simulink library "ParsingLibrary"  (Simulink 8.2)
settings: Solver=ode45  StartTime=0.0  StopTime=10.0  RelTol=1e-3
undefined symbols (not defined in the file): Indicies
libraries: simulink x1
settings Model: Creator=Scott  LastModifiedBy=leidos

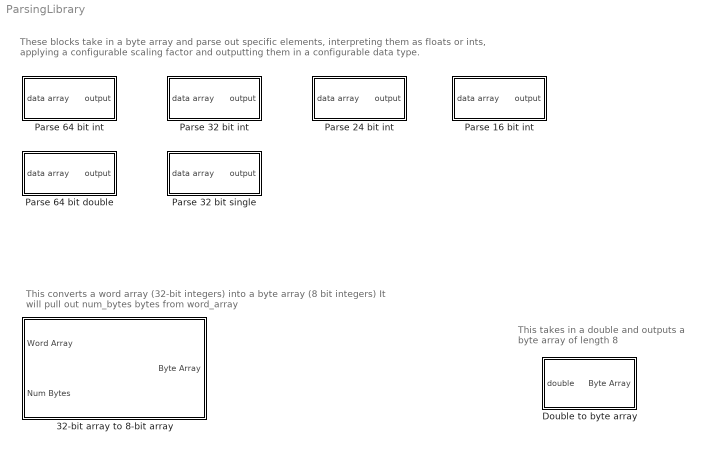
== system ParsingLibrary ==
  note: This takes in a double and outputs
      | a byte array of length 8
  note: This converts a word array (32-bit integers) into a byte array (8 bit integers)
      | It will pull out num_bytes bytes from word_array
  note: These blocks take in a byte array and parse out specific elements, interpreting them as floats or ints, applying
      | a configurable scaling factor and outputting them in a configurable data type.
  32-bit array to 8-bit array : Subsystem  TreatAsAtomicUnit=on
  "Double to byte array " : Subsystem  TreatAsAtomicUnit=on
  Parse 16 bit int : Subsystem  mask{Value=[0:1], InDataTypeStr=uint16, factor=1, OutDataTypeStr=single}
      mask prompts: Value "Elements to parse:"; InDataTypeStr "Interpret data as:"; factor "Scaling factor:"; OutDataTypeStr "Output data type:"
      mask TypeOptions Value: Constant/Value
      mask TypeOptions InDataTypeStr: Input Type/OutDataTypeStr
      mask TypeOptions factor: Factor/Value
      mask TypeOptions OutDataTypeStr: multiply/OutDataTypeStr
  Parse 24 bit int : Subsystem  mask{Value2=[0:2], OutDataTypeStr=double, InDataTypeStr=int32, Value=1}
      mask prompts: Value2 "Elements to parse:"; OutDataTypeStr "Output data type:"; InDataTypeStr "Interpret data as:"; Value "Scale Factor:"
      mask TypeOptions Value2: Constant/Value
      mask TypeOptions OutDataTypeStr: multiply/OutDataTypeStr
      mask TypeOptions InDataTypeStr: Input Type/OutDataTypeStr
      mask TypeOptions Value: Factor/Value
  Parse 32 bit int : Subsystem  mask{Value2=[0:3], OutDataTypeStr=double, InDataTypeStr=uint32, Value=1}
      mask prompts: Value2 "Elements to parse:"; OutDataTypeStr "Output data type:"; InDataTypeStr "Interpret data as:"; Value "Scale Factor:"
      mask TypeOptions Value2: Constant/Value
      mask TypeOptions OutDataTypeStr: multiply/OutDataTypeStr
      mask TypeOptions InDataTypeStr: Input Type/OutDataTypeStr
      mask TypeOptions Value: Factor/Value
  Parse 32 bit single : Subsystem  mask{Value=Indicies, Flip=true, factor=1, OutDataTypeStr=single}
      mask prompts: Value "Indicies:"; Flip "Flip Bytes?:"; factor "Scale Factor:"; OutDataTypeStr "Output data type:"
      mask TypeOptions Value: Constant/Value
      mask TypeOptions Flip: Constant1/Value
      mask TypeOptions factor: Factor/Value
      mask TypeOptions OutDataTypeStr: multiply/OutDataTypeStr
  Parse 64 bit double : Subsystem  mask{Value=[0:7], factor=1, OutDataTypeStr=double}
      mask prompts: Value "Index"; factor "Scale Factor:"; OutDataTypeStr "Output data type:"
      mask TypeOptions Value: Selector/Indices
      mask TypeOptions factor: Factor/Value
      mask TypeOptions OutDataTypeStr: multiply/OutDataTypeStr
  Parse 64 bit int : Subsystem  mask{Value=[0:7], factor=1, OutDataTypeStr=double}
      mask prompts: Value "Indicies:"; factor "Scale factor:"; OutDataTypeStr "Output data type:"
      mask TypeOptions Value: Constant/Value
      mask TypeOptions factor: Factor/Value
      mask TypeOptions OutDataTypeStr: multiply/OutDataTypeStr

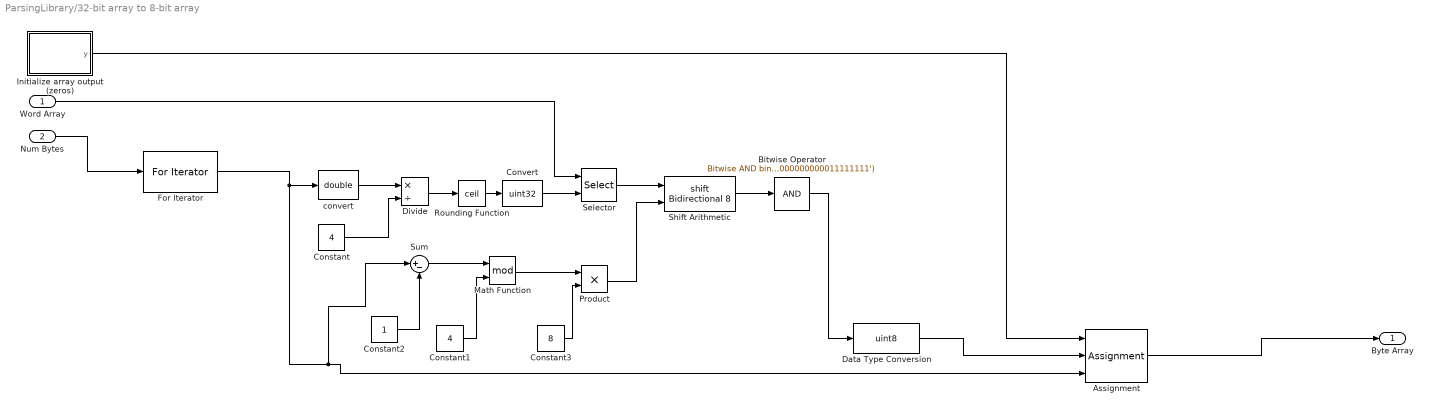
== system ParsingLibrary/32-bit array to 8-bit array ==
  Word Array : Inport  OutDataTypeStr=uint32
  Num Bytes : Inport  Port=2
  Assignment : Assignment  IndexOptions=Index vector (port)  Indices=1  OutputSizes=[1 1]
  Bitwise Operator : simulink/Logic and Bit Operations/Bitwise Operator  logicop=AND  UseBitMask=on  BitMask=bin2dec('00000000000000000000000011111111')  BitMaskRealWorld=Stored Integer
  Constant : Constant  Value=4  OutDataTypeStr=double
  Constant1 : Constant  Value=4  OutDataTypeStr=int32
  Constant2 : Constant  OutDataTypeStr=int32
  Constant3 : Constant  Value=8  OutDataTypeStr=int32
  Convert : DataTypeConversion  OutDataTypeStr=uint32
  Data Type Conversion : DataTypeConversion  OutDataTypeStr=uint8
  Divide : Product  Inputs=*/
  For Iterator : ForIterator  ResetStates=reset  IterationSource=external  IterationLimit=6
  Initialize array output (zeros) : MATLAB Function  TreatAsAtomicUnit=on
  Math Function : Math  Operator=mod  SaturateOnIntegerOverflow=on
  Product : Product  OutDataTypeStr=uint32
  Rounding Function : Rounding  Operator=ceil
  Selector : Selector  IndexOptions=Index vector (port)  Indices=[1 3]  OutputSizes=1
  Shift Arithmetic : ArithShift  BitShiftNumberSource=Input port  BitShiftNumber=8  DiagnosticForOORShift=Warning  CheckOORBitShift=on
      settings: InputPortMap=u0,p1
  Sum : Sum  Inputs=|+-  OutDataTypeStr=int32
  convert : DataTypeConversion  OutDataTypeStr=double
  Byte Array : Outport
  wires:
  Initialize array output (zeros)/1(y) -> Assignment/1
  Selector/1 -> Shift Arithmetic/1
  For Iterator/1 -> Sum/1, Assignment/3, convert/1
  Constant/1 -> Divide/2
  Divide/1 -> Rounding Function/1
  Word Array/1 -> Selector/1
  Constant1/1 -> Math Function/2
  Constant3/1 -> Product/2
  Product/1 -> Shift Arithmetic/2
  Shift Arithmetic/1 -> Bitwise Operator/1
  Bitwise Operator/1 -> Data Type Conversion/1
  Data Type Conversion/1 -> Assignment/2
  Num Bytes/1 -> For Iterator/1
  convert/1 -> Divide/1
  Rounding Function/1 -> Convert/1
  Convert/1 -> Selector/2
  Math Function/1 -> Product/1
  Constant2/1 -> Sum/2
  Sum/1 -> Math Function/1
  Assignment/1 -> Byte Array/1

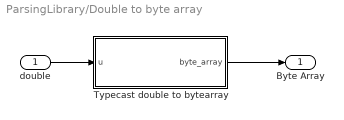
== system ParsingLibrary/Double to byte array  ==
  double : Inport  OutDataTypeStr=double
  Typecast double to bytearray : MATLAB Function  TreatAsAtomicUnit=on
  Byte Array : Outport  OutDataTypeStr=uint8
  wires:
  double/1 -> Typecast double to bytearray/1(u)
  Typecast double to bytearray/1(byte_array) -> Byte Array/1

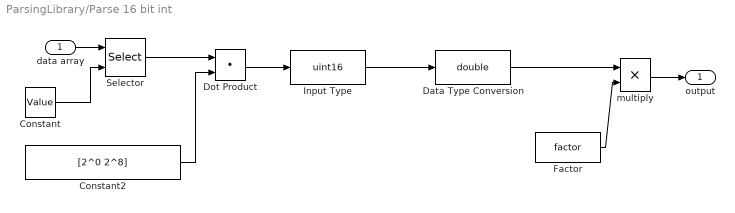
== system ParsingLibrary/Parse 16 bit int ==
  data array : Inport
  Constant : Constant  Value=Value  OutDataTypeStr=uint32
  Constant2 : Constant  Value=[2^0 2^8]  OutDataTypeStr=uint32
  Data Type Conversion : DataTypeConversion  OutDataTypeStr=double
  Dot Product : DotProduct  OutDataTypeStr=uint16
  Factor : Constant  Value=factor  OutDataTypeStr=double
  Input Type : DataTypeConversion  OutDataTypeStr=uint16
  Selector : Selector  IndexMode=Zero-based  IndexOptions=Index vector (port)  Indices=[0:1]  OutputSizes=1
  multiply : Product  Inputs=**  OutDataTypeStr=single
  output : Outport
  wires:
  multiply/1 -> output/1
  Factor/1 -> multiply/2
  Dot Product/1 -> Input Type/1
  Constant2/1 -> Dot Product/2
  data array/1 -> Selector/1
  Selector/1 -> Dot Product/1
  Input Type/1 -> Data Type Conversion/1
  Data Type Conversion/1 -> multiply/1
  Constant/1 -> Selector/2

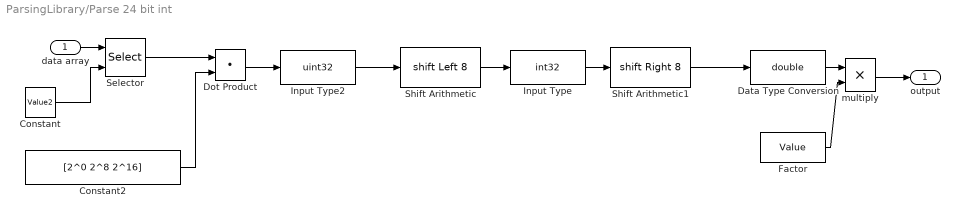
== system ParsingLibrary/Parse 24 bit int ==
  data array : Inport
  Constant : Constant  Value=Value2  OutDataTypeStr=uint32
  Constant2 : Constant  Value=[2^0 2^8 2^16]  OutDataTypeStr=uint32
  Data Type Conversion : DataTypeConversion  OutDataTypeStr=double
  Dot Product : DotProduct  OutDataTypeStr=uint32
  Factor : Constant  Value=Value  OutDataTypeStr=double
  Input Type : DataTypeConversion  OutDataTypeStr=int32  ConvertRealWorld=Stored Integer (SI)
  Input Type2 : DataTypeConversion  OutDataTypeStr=uint32  ConvertRealWorld=Stored Integer (SI)
  Selector : Selector  IndexMode=Zero-based  IndexOptions=Index vector (port)  Indices=[0:3]  OutputSizes=1
  Shift Arithmetic : ArithShift  BitShiftNumber=8  BitShiftDirection=Left
  Shift Arithmetic1 : ArithShift  BitShiftNumber=8  BitShiftDirection=Right
  multiply : Product  Inputs=**  OutDataTypeStr=double
  output : Outport
  wires:
  multiply/1 -> output/1
  Factor/1 -> multiply/2
  Constant2/1 -> Dot Product/2
  data array/1 -> Selector/1
  Selector/1 -> Dot Product/1
  Data Type Conversion/1 -> multiply/1
  Constant/1 -> Selector/2
  Shift Arithmetic1/1 -> Data Type Conversion/1
  Dot Product/1 -> Input Type2/1
  Input Type2/1 -> Shift Arithmetic/1
  Shift Arithmetic/1 -> Input Type/1
  Input Type/1 -> Shift Arithmetic1/1

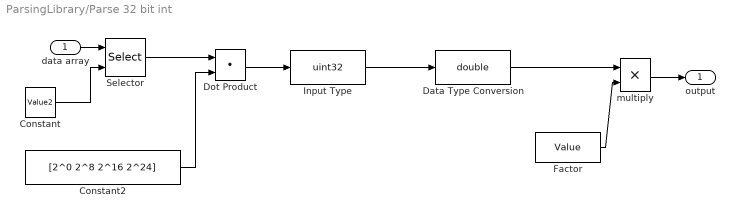
== system ParsingLibrary/Parse 32 bit int ==
  data array : Inport
  Constant : Constant  Value=Value2  OutDataTypeStr=uint32
  Constant2 : Constant  Value=[2^0 2^8 2^16 2^24]  OutDataTypeStr=uint32
  Data Type Conversion : DataTypeConversion  OutDataTypeStr=double
  Dot Product : DotProduct  OutDataTypeStr=uint32
  Factor : Constant  Value=Value  OutDataTypeStr=double
  Input Type : DataTypeConversion  OutDataTypeStr=uint32  ConvertRealWorld=Stored Integer (SI)
  Selector : Selector  IndexMode=Zero-based  IndexOptions=Index vector (port)  Indices=[0:3]  OutputSizes=1
  multiply : Product  Inputs=**  OutDataTypeStr=double
  output : Outport
  wires:
  multiply/1 -> output/1
  Factor/1 -> multiply/2
  Dot Product/1 -> Input Type/1
  Constant2/1 -> Dot Product/2
  data array/1 -> Selector/1
  Selector/1 -> Dot Product/1
  Input Type/1 -> Data Type Conversion/1
  Data Type Conversion/1 -> multiply/1
  Constant/1 -> Selector/2

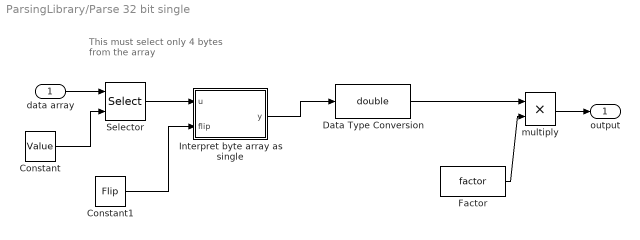
== system ParsingLibrary/Parse 32 bit single ==
  note: This must select
      | only 4 bytes from
      | the array
  data array : Inport
  Constant : Constant  Value=Value  OutDataTypeStr=uint32
  Constant1 : Constant  Value=Flip  OutDataTypeStr=boolean
  Data Type Conversion : DataTypeConversion  OutDataTypeStr=double
  Factor : Constant  Value=factor  OutDataTypeStr=double
  Interpret byte array as single : MATLAB Function  TreatAsAtomicUnit=on
  Selector : Selector  IndexMode=Zero-based  IndexOptions=Index vector (port)  Indices=[0:3]  OutputSizes=1
  multiply : Product  Inputs=**  OutDataTypeStr=single
  output : Outport
  wires:
  data array/1 -> Selector/1
  Factor/1 -> multiply/2
  multiply/1 -> output/1
  Selector/1 -> Interpret byte array as single/1(u)
  Interpret byte array as single/1(y) -> Data Type Conversion/1
  Data Type Conversion/1 -> multiply/1
  Constant/1 -> Selector/2
  Constant1/1 -> Interpret byte array as single/2(flip)

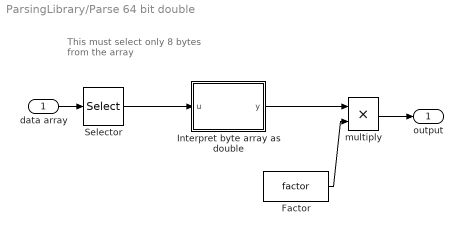
== system ParsingLibrary/Parse 64 bit double ==
  note: This must select
      | only 8 bytes from
      | the array
  data array : Inport
  Factor : Constant  Value=factor  OutDataTypeStr=double
  Interpret byte array as double : MATLAB Function  TreatAsAtomicUnit=on
  Selector : Selector  IndexMode=Zero-based  IndexOptions=Index vector (dialog)  Indices=[0:7]  OutputSizes=1
  multiply : Product  Inputs=**  OutDataTypeStr=double
  output : Outport
  wires:
  multiply/1 -> output/1
  Factor/1 -> multiply/2
  data array/1 -> Selector/1
  Selector/1 -> Interpret byte array as double/1(u)
  Interpret byte array as double/1(y) -> multiply/1

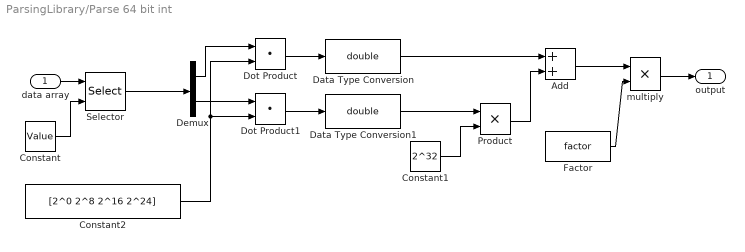
== system ParsingLibrary/Parse 64 bit int ==
  data array : Inport
  Add : Sum  AccumDataTypeStr=double
  Constant : Constant  Value=Value  OutDataTypeStr=uint32
  Constant1 : Constant  Value=2^32  OutDataTypeStr=double
  Constant2 : Constant  Value=[2^0 2^8 2^16 2^24]  OutDataTypeStr=uint32
  Data Type Conversion : DataTypeConversion  OutDataTypeStr=double
  Data Type Conversion1 : DataTypeConversion  OutDataTypeStr=double
  Demux : Demux  Outputs=2
  Dot Product : DotProduct  OutDataTypeStr=Inherit: Inherit via internal rule
  Dot Product1 : DotProduct  OutDataTypeStr=Inherit: Inherit via internal rule
  Factor : Constant  Value=factor  OutDataTypeStr=double
  Product : Product  OutDataTypeStr=double  RndMeth=Zero
  Selector : Selector  IndexMode=Zero-based  IndexOptions=Index vector (port)  Indices=[0:7]  OutputSizes=1
  multiply : Product  Inputs=**  OutDataTypeStr=double
  output : Outport
  wires:
  data array/1 -> Selector/1
  Selector/1 -> Demux/1
  Constant2/1 -> Dot Product/2, Dot Product1/2
  Constant1/1 -> Product/2
  Data Type Conversion1/1 -> Product/1
  Product/1 -> Add/2
  Data Type Conversion/1 -> Add/1
  Dot Product1/1 -> Data Type Conversion1/1
  Dot Product/1 -> Data Type Conversion/1
  Demux/2 -> Dot Product1/1
  Demux/1 -> Dot Product/1
  Add/1 -> multiply/1
  Factor/1 -> multiply/2
  multiply/1 -> output/1
  Constant/1 -> Selector/2

== matlab function Parse 64 bit double/Interpret byte array as double ==
  data: u input double; y output double
function y = fcn(u)
%#codegen
y = double(0.0);

y = typecast(flipud(uint8(u)), 'double');

== matlab function Parse 32 bit single/Interpret byte array as single ==
  data: u input double; y output double; flip input double
function y = fcn(u, flip)
%#codegen
y = single(0.0);

if (flip)
    u = fliplr(u);
end
y = typecast(uint8(u), 'single');

== matlab function Double to byte array /Typecast double to bytearray ==
  data: u input double; byte_array output double
function byte_array = fcn(u)
%#codegen
byte_array = zeros(1,8, 'uint8');
byte_array = typecast(u, 'uint8');

== matlab function 32-bit array to 8-bit array/Initialize array output (zeros) ==
  data: y output double
function y = fcn()
%#codegen

y = zeros(1,1472, 'uint8');
